simulink model "QuadSimulationVrepHoverDIV5"  (R2013a)
settings: Solver=ode1  StartTime=0  StopTime=10  FixedStep=0.01  MaxStep=0.06  RelTol=1e-3
model workspace (MAT data in the model file):
  Sig = Simulink.Signal
  Sig.DataType = 'auto'
  Sig.Dimensions = -1
  Sig.DimensionsMode = 'auto'
  Sig.Complexity = 'auto'
  Sig.SampleTime = -1
  Sig.SamplingMode = 'auto'
values from neighbouring files (symbols this model uses):
  IC = struct('P',(P),'Q',(Q),'R',(R),'Phi',(Phi),'The',(The),'Psi',(Psi),     'U',(U),'V',(V),'W',(W),'X',(X),'Y',(Y),'Z',(Z),'w1',(w1),'w2',(w2),'w3',(w3),'w4',(w4))    [ICgen.m]    (also in quadcopterDynamicsSFunction.m = block.DialogPrm(2).Data; quadcopterDynamicsSFunctionVrepV4.m = block.DialogPrm(2).Data; quadcopterDynamicsSFunctionVrepV5.m = block.DialogPrm(2).Data; quadcopterDynamicsSFunctionVrepV6.m = block.DialogPrm(2).Data)
  quadModel = struct('g',(g),'d',(d),'mass',(mass),'ct',(ct),'cq',(cq),     'Jx',(Jx),'Jy',(Jy),'Jz',(Jz),'Jm',(Jm),'Jb',(Jb),'Jbinv',(Jbinv),'dctcq',(dctcq),     'motor_m',(motor_m),'motor_dm',(motor_dm),'motor_h',(motor_h),'motor_r',(motor_r),     'ESC_m',(ESC_m),'ESC_a',(ESC_a),'ESC_b',(ESC_b),'ESC_ds',(ESC_ds),     'HUB_m',(HUB_m),'HUB_r',(HUB_r),'HUB_H',(HUB_H),     'arms_m',(arms_m),'arms_r',(arms_r),'arm ...(+111 chars)    [ModelGen.m]
undefined symbols (not defined in the file or in its folder): DiscIntNeverNeededParam, sigbuilder_block
libraries: simulink x7
Description:
  | This is a configurable quadcopter simulation.
  | This Simulink model demonstates attitude control.
  | 
  | Additional quadcopter modeling and simulation materials available at:
  | github.com/dch33/Quad-Sim
  | 
  | Copyright (C) 2014 D. Hartman, K. Landis, S. Moreno, J. Kim, M. Mehrer
  | 
  | License:
  |     This program is free software: you can redistribute it and/or modify
  |     it under the terms of the GNU LESSER GENERAL PUBLIC LICENSE as published by
  |     the Free Software Foundation, either version 3 of the License, or
  |     (at your option) any later version.
  | 
  |     This program is distributed in the hope that it will be useful,
  |     but WITHOUT ANY WARRANTY; without even the implied warranty of
  |     MERCHANTABILITY or FITNESS FOR A PARTICULAR PURPOSE.  See the
  |     GNU General Public License for more details.
  | 
  |     You should have received a copy of the GNU LESSER GENERAL PUBLIC LICENSE
  |     along with this program.  If not, see <http://www.gnu.org/licenses/>.
settings Model: ModifiedComment=Javid -- Tue Dec 01 00:24:24 2015 -- Version 1.43  Creator=David Hartman  LastModifiedBy=Javid
settings Model: ModifiedHistory=|
  | Javid -- Tue Dec 01 00:24:24 2015 -- Version 1.43
  | 
  | 
  | Javid -- Tue Dec 01 00:24:24 2015 -- Version 1.43
  | 
  | 
  | Javid -- Mon Nov 30 23:34:52 2015 -- Version 1.40
  | 
  | 
  | Javid -- Mon Nov 30 23:34:54 2015 -- Version 1.41
  | 
  | 
  | Javid -- Mon Nov 30 23:34:52 2015 -- Version 1.40
  | 
  | 
  | Cavid -- Mon Nov 30 13:04:43 2015 -- Version 1.39
  | 
  | 
  | Cavid -- Mon Nov 30 13:00:14 2015 -- Version 1.38
  | 
  | 
  | Javid -- Mon Nov 30 00:31:13 2015 -- Version 1.37
  | 
  | 
  | Javid -- Sun Nov 29 23:37:43 2015 -- Version 1.36
  | 
  | 
  | Javid -- Sun Nov 29 22:57:34 2015 -- Version 1.35
  | 
  | 
  | Javid -- Sun Nov 29 15:59:30 2015 -- Version 1.34
  | 
  | 
  | Javid -- Thu Nov 19 09:09:11 2015 -- Version 1.33
  | 
  | 
  | Javid -- Thu Nov 19 02:22:34 2015 -- Version 1.32
  | 
  | 
  | Javid -- Thu Nov 19 02:17:10 2015 -- Version 1.31
  | 
  | 
  | Javid -- Thu Nov 19 01:41:29 2015 -- Version 1.30
  | 
  | 
  | Javid -- Thu Nov 19 01:37:38 2015 -- Version 1.29
  | 
  | 
  | Javid -- Thu Nov 19 00:11:49 2015 -- Version 1.28
  | 
  | 
  | Javid -- Wed Nov 18 23:13:28 2015 -- Version 1.27
  | 
  | 
  | Javid -- Wed Nov 18 22:55:25 2015 -- Version 1.26
  | 
  | 
  | Javid -- Wed Nov 18 22:55:20 2015 -- Version 1.25
  | 
  | 
  | Javid -- Wed Nov 18 22:55:20 2015 -- Version 1.25
  | 
  | 
  | Javid -- Tue Nov 17 23:07:53 2015 -- Version 1.24
  | 
  | 
  | Javid -- Tue Nov 17 22:43:13 2015 -- Version 1.23
  | 
  | 
  | Javid -- Tue Nov 17 22:37:48 2015 -- Version 1.22
  | 
  | 
  | Javid -- Tue Nov 17 22:19:46 2015 -- Version 1.21
  | 
  | 
  | Javid -- Sun Nov 15 18:42:45 2015 -- Version 1.20
  | 
  | 
  | Javid -- Sat Nov 14 16:44:47 2015 -- Version 1.19
  | 
  | 
  | Cavid -- Mon Nov 09 15:07:19 2015 -- Version 1.18
  | 
  | 
  | Cavid -- Mon Nov 09 12:56:30 2015 -- Version 1.17
  | 
  | 
  | Javid -- Thu Nov 05 21:32:59 2015 -- Version 1.16
  | 
  | 
  | Javid -- Thu Nov 05 00:31:36 2015 -- Version 1.14
  | 
  | 
  | Javid -- Thu Nov 05 00:31:37 2015 -- Version 1.14
  | 
  | 
  | Javid -- Wed Nov 04 23:11:59 2015 -- Version 1.13
  | 
  | 
  | Javid -- Sat Oct 31 23:55:35 2015 -- Version 1.12
  | 
  | 
  | Javid -- Sat Oct 31 20:30:45 2015 -- Version 1.11
  | 
  | 
  | Cavid -- Mon Oct 19 16:53:56 2015 -- Version 1.10
  | 
  | 
  | Cavid -- Mon Oct 19 11:55:21 2015 -- Version 1.9
  | 
  | 
  | Cavid -- Mon Oct 19 11:50:10 2015 -- Version 1.8
  | 
  | 
  | Cavid -- Mon Oct 19 11:48:50 2015 -- Version 1.7
  | 
  | 
  | Cavid -- Mon Oct 19 11:27:32 2015 -- Version 1.6
  | 
  | 
  | davidhartman -- Fri Jun 06 23:19:51 2014 -- Version 1.5
  | 
  | 
  | davidhartman -- Fri Jun 06 22:53:10 2014 -- Version 1.3
settings SolverCC: AutoInsertRateTranBlk=on
settings DataIOCC: LimitDataPoints=off  SignalLogging=off
settings OptimizationCC: InlineParams=on
settings DebuggingCC: UniqueDataStoreMsg=warning  StrictBusMsg=WarnOnBusTreatedAsVector

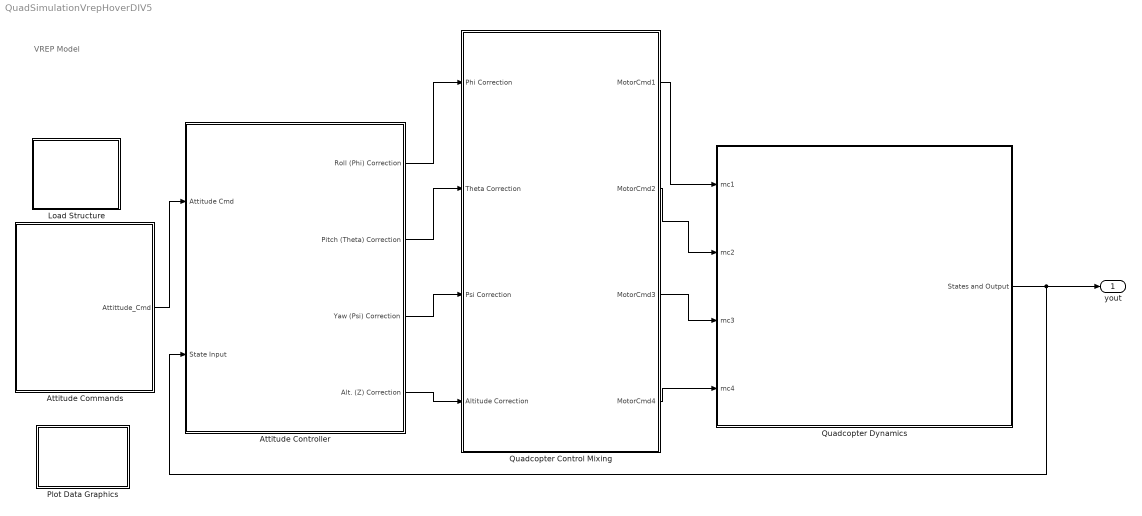
== system QuadSimulationVrepHoverDIV5 ==
  note: VREP Model
  Attitude Commands : Subsystem
  Attitude Controller : Subsystem
  Load Structure : Subsystem
      settings: OpenFcn=|
      | uiopen('load')
      | if (exist('IC')==1 && exist('quadModel')==1)
      | set_param(bdroot, 'SimulationCommand', 'update')
      | end
      mask Display: fprintf('LOAD:\nModel and\nIC\n');
  Plot Data Graphics : Subsystem
      settings: OpenFcn=|
      | if exist('yout')
      | yout = evalin('base', 'yout');
      | tout = evalin('base', 'tout');
      | quadPlotsV3(yout, tout)
      | else
      | msgbox('Simulation must be run before data can be plotted.')
      | end
      mask Display: fprintf('Plots')
  Quadcopter Control Mixing : Subsystem
      mask Display:
      | modelLoaded = evalin('base','exist(''quadModel'',''var'')');
      | if (modelLoaded==1)
      |     if (evalin('base','quadModel.plusConfig'))
      |     fprintf([' \n' ' \n'  'Configuration "+"']);
      |     else if (~evalin('base','quadModel.plusConfig'))
      |         fprintf([' \n' ' \n' 'Configuration "X"']);
      |         end
      |     end
      | else
      |     fprintf([' \n' ' \n'  'Model Not Loaded']);
      | end
  Quadcopter Dynamics : Subsystem
  yout : Outport
  wires:
  Quadcopter Control Mixing/1(MotorCmd1) -> Quadcopter Dynamics/1(mc1)
  Quadcopter Control Mixing/2(MotorCmd2) -> Quadcopter Dynamics/2(mc2)
  Quadcopter Control Mixing/3(MotorCmd3) -> Quadcopter Dynamics/3(mc3)
  Quadcopter Control Mixing/4(MotorCmd4) -> Quadcopter Dynamics/4(mc4)
  Attitude Controller/1(Roll (Phi) Correction) -> Quadcopter Control Mixing/1(Phi Correction)
  Attitude Controller/2(Pitch (Theta) Correction) -> Quadcopter Control Mixing/2(Theta Correction)
  Attitude Controller/3(Yaw (Psi) Correction) -> Quadcopter Control Mixing/3(Psi Correction)
  Attitude Controller/4(Alt. (Z) Correction) -> Quadcopter Control Mixing/4(Altitude Correction)
  Attitude Commands/1(Attittude_Cmd) -> Attitude Controller/1(Attitude Cmd)
  Quadcopter Dynamics/1(States and Output) -> Attitude Controller/2(State Input), yout/1

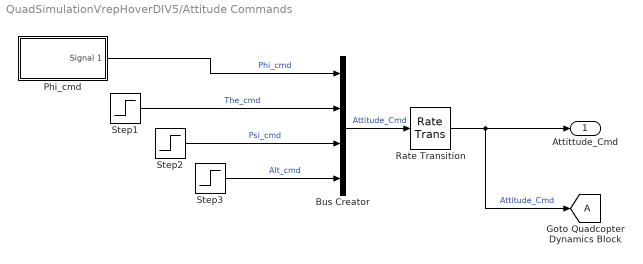
== system QuadSimulationVrepHoverDIV5/Attitude Commands ==
  Bus Creator : BusCreator
  Phi_cmd : Subsystem  Tag=STV Subsys  LoadFcn=sigbuilder_block('load');  StartFcn=sigbuilder_block('start');  StopFcn=sigbuilder_block('stop');  ClipboardFcn=sigbuilder_block('clipboard');  mask(Sigbuilder block){}
      mask help: Simulink:masks:SigbuilderBlock_MD
      mask init:
      | if ~strcmp(get_param(bdroot(gcbh),'SimulationStatus'),'stopped') tuvar = sigbuilder_block('maskInit'); end
      settings: CopyFcn=sigbuilder_block('copy');  DeleteFcn=sigbuilder_block('delete');  ModelCloseFcn=sigbuilder_block('modelClose');  PreSaveFcn=sigbuilder_block('preSave');  PauseFcn=sigbuilder_block('pause');  ContinueFcn=sigbuilder_block('continue');  NameChangeFcn=sigbuilder_block('namechange');  OpenFcn=sigbuilder_block('open',[6.75 6.75 1138.5 568.5 ]);  CloseFcn=sigbuilder_block('close');
      mask Display: plot(0, 0, 100, 100,[2, 2, 32, 32, 2], [68, 8, 8, 68, 68],[32, 2], [38, 38], [32, 19, 2],[53, 60, 44], [32, 17, 17, 2],[16, 16, 31, 31]);txt = getActiveGroup(gcbh);text(2, 100, txt,'verticalAlignment', 'top');
  Rate Transition : RateTransition  Deterministic=off  OutPortSampleTime=0.01
  Step1 : Step  Time=0  After=0  SampleTime=0
  Step2 : Step  Time=0  Before=-pi/2  After=-pi/2  SampleTime=0
  Step3 : Step  Time=0  Before=1.5  After=1.5  SampleTime=0
  Attittude_Cmd : Outport
  tag scope: A=global
  wires:
  Step3/1 -> Bus Creator/4  "Alt_cmd"
  Step2/1 -> Bus Creator/3  "Psi_cmd"
  Step1/1 -> Bus Creator/2  "The_cmd"
  Phi_cmd/1(Signal 1) -> Bus Creator/1  "Phi_cmd"
  Bus Creator/1 -> Rate Transition/1  "Attitude_Cmd"
  Rate Transition/1 -> [A], Attittude_Cmd/1  "Attitude_Cmd"

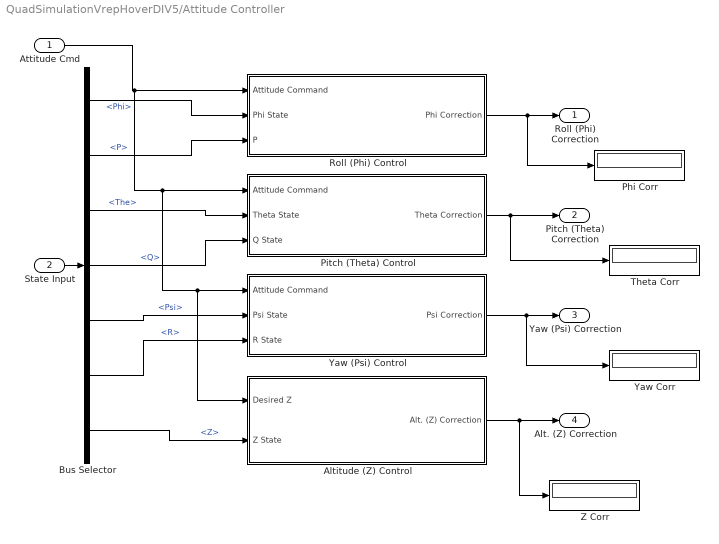
== system QuadSimulationVrepHoverDIV5/Attitude Controller ==
  Attitude Cmd : Inport
  State Input : Inport  Port=2
  Altitude (Z) Control : Subsystem  mask{Kpz=16, Kiz=1, Kdz=10, LimitOutput=on, USat=1, LSat=-1, GOffset=(sqrt((quadModel.mass*quadModel.g)/(4*quadModel.ct))-quadModel.b)/quadModel.cr}
      mask prompts: Kpz "Kp"; Kiz "Ki"; Kdz "Kd"; LimitOutput "Integral Saturation?"; USat "Upper saturation limit:"; LSat "Lower saturation limit:"; GOffset "Gravity Feedforward"
      mask help:
      | Adjust PID controller gains through this mask interface, or "look under mask" for more detailed adjustments.
      |
      | Note: Gravity Offset will not appear on block face as a value until simulation is run if it is the result of a formula involving the quadcopter model parameters.
      mask TypeOptions Kpz: Kpz/Gain
      mask TypeOptions Kiz: Kiz/Gain
      mask TypeOptions Kdz: Kdz/Gain
      mask TypeOptions LimitOutput:
      | Integrator
      | Limited/LimitOutput
      mask TypeOptions USat:
      | Integrator
      | Limited/UpperSaturationLimit
      mask TypeOptions LSat:
      | Integrator
      | Limited/LowerSaturationLimit
      mask TypeOptions GOffset: Gravity Offset (Level Flight)/Value
      mask Display:
      | fprintf(['Gravity Offset = ' num2str(GOffset) '\n' ...
      |     'Kp = ' num2str(Kpz) '\n' ...
      |     'Ki = ' num2str(Kiz) '\n' ...
      |     'Kd = ' num2str(Kdz) '\n' ...
      |     'Integral Saturation: ' LimitOutput]);
      | if strcmp(LimitOutput,'on')
      |     fprintf([' \n' ' \n' ' \n' ' \n' ' \n' '\n' ...
      |         'Limits: ' num2str(USat) ' to ' num2str(LSat)]);
      | end
  Bus Selector : BusSelector  OutputSignals=Phi,P,The,Q,Psi,R,Z
  Phi Corr : Display
  Pitch (Theta) Control : Subsystem  mask{Kpt=25, Kit=0, Kdt=6, Kdt2=0, LimitOutput=on, USat=10, LSat=-10}
      mask prompts: Kpt "Kp"; Kit "Ki"; Kdt "Kd"; Kdt2 "Kd2"; LimitOutput "Integral Saturation?"; USat "Upper saturation limit:"; LSat "Lower saturation limit:"
      mask help: Adjust PID controller gains through this mask interface, or "look under mask" for more detailed adjustments.
      mask TypeOptions Kpt: Kpt/Gain
      mask TypeOptions Kit: Kit/Gain
      mask TypeOptions Kdt: Kdt/Gain
      mask TypeOptions Kdt2: Kdt2/Gain
      mask TypeOptions LimitOutput:
      | Discrete-Time
      | Integrator/LimitOutput
      mask TypeOptions USat:
      | Discrete-Time
      | Integrator/UpperSaturationLimit
      mask TypeOptions LSat:
      | Discrete-Time
      | Integrator/LowerSaturationLimit
      mask Display:
      | % port_label('input',1,'Theta Command');
      | % port_label('input',2,'Theta State');
      | % port_label('input',3,'Q State');
      | % port_label('output',1,'Theta Correction');
      | fprintf(['Kp = ' num2str(Kpt) '\n' ...
      |     'Ki = ' num2str(Kit) '\n' ...
      |     'Kd = ' num2str(Kdt) '\n' ...
      |     'Kd2= ' num2str(Kdt2) '\n' ...
      |     'Integral Saturation: ' LimitOutput]);
      | if strcmp(LimitOutput,'on')
      |     fprintf([' \n' ' \n' ' \n' ' \n' '\n' '\n' ...
      |         'Limits: ' num2str(USat) ' to ' num2str(LSat)]);
      | end
  "Roll (Phi) Control " : Subsystem  mask{Kpp=25, Kip=0, Kdp=6, Kdp2=0, LimitOutput=on, USat=10, LSat=-10}
      mask prompts: Kpp "Kp"; Kip "Ki"; Kdp "Kd"; Kdp2 "Kd2"; LimitOutput "Integral Saturation:"; USat "Upper saturation limit:"; LSat "Lower saturation limit:"
      mask help:
      | Adjust PID controller gains through this mask interface, or "look under mask"
      | for more detailed adjustments.
      mask TypeOptions Kpp: Kpp/Gain
      mask TypeOptions Kip: Kip/Gain
      mask TypeOptions Kdp: Kdp/Gain
      mask TypeOptions Kdp2: Kdp2/Gain
      mask TypeOptions LimitOutput:
      | Discrete-Time
      | Integrator/LimitOutput
      mask TypeOptions USat:
      | Discrete-Time
      | Integrator/UpperSaturationLimit
      mask TypeOptions LSat:
      | Discrete-Time
      | Integrator/LowerSaturationLimit
      mask Display:
      | fprintf(['Kp = ' num2str(Kpp) '\n' ...
      |     'Ki = ' num2str(Kip) '\n' ...
      |     'Kd = ' num2str(Kdp) '\n'...
      |     'Kd2= ' num2str(Kdp2) '\n'...
      |     'Integral Saturation: ' LimitOutput]);
      | if strcmp(LimitOutput,'on')
      |     fprintf([' \n' ' \n' ' \n' ' \n' '\n' '\n' ...
      |         'Limits: ' num2str(USat) ' to ' num2str(LSat)]);
      | end
  Theta Corr : Display
  Yaw (Psi) Control : Subsystem  mask{Kps=0, Kis=0, Kds=0, Kds2=0, LimitOutput=on, USat=1, LSat=-1}
      mask prompts: Kps "Kp"; Kis "Ki"; Kds "Kd"; Kds2 "Kd2"; LimitOutput "Integral Saturation?"; USat "Upper saturation limit:"; LSat "Lower saturation limit:"
      mask help: Adjust PID controller gains through this mask interface, or "look under mask" for more detailed adjustments.
      mask TypeOptions Kps: Kps/Gain
      mask TypeOptions Kis: Kit/Gain
      mask TypeOptions Kds: Kds/Gain
      mask TypeOptions Kds2: Kds2/Gain
      mask TypeOptions LimitOutput:
      | Discrete-Time
      | Integrator/LimitOutput
      mask TypeOptions USat:
      | Discrete-Time
      | Integrator/UpperSaturationLimit
      mask TypeOptions LSat:
      | Discrete-Time
      | Integrator/LowerSaturationLimit
      mask Display:
      | fprintf(['Kp = ' num2str(Kps) '\n' ...
      |     'Ki = ' num2str(Kis) '\n' ...
      |     'Kd = ' num2str(Kds) '\n' ...
      |     'Kd2 = ' num2str(Kds2) '\n' ...
      |     'Integral Saturation: ' LimitOutput]);
      | if strcmp(LimitOutput,'on')
      |     fprintf([' \n' ' \n' ' \n' ' \n' '\n' '\n' ...
      |         'Limits: ' num2str(USat) ' to ' num2str(LSat)]);
      | end
  Yaw Corr : Display
  Z Corr : Display
  Roll (Phi) Correction : Outport
  Pitch (Theta) Correction : Outport  Port=2
  Yaw (Psi) Correction : Outport  Port=3
  Alt. (Z) Correction : Outport  Port=4
  wires:
  Bus Selector/6 -> Yaw (Psi) Control/3(R State)  "<R>"
  Bus Selector/4 -> Pitch (Theta) Control/3(Q State)  "<Q>"
  Bus Selector/2 -> "Roll (Phi) Control "/3(P)  "<P>"
  Bus Selector/3 -> Pitch (Theta) Control/2(Theta State)  "<The>"
  Bus Selector/7 -> Altitude (Z) Control/2(Z State)  "<Z>"
  Bus Selector/5 -> Yaw (Psi) Control/2(Psi State)  "<Psi>"
  Yaw (Psi) Control/1(Psi Correction) -> Yaw Corr/1, Yaw (Psi) Correction/1
  Pitch (Theta) Control/1(Theta Correction) -> Theta Corr/1, Pitch (Theta) Correction/1
  Bus Selector/1 -> "Roll (Phi) Control "/2(Phi State)  "<Phi>"
  "Roll (Phi) Control "/1(Phi Correction) -> Phi Corr/1, Roll (Phi) Correction/1
  Altitude (Z) Control/1(Alt. (Z) Correction) -> Z Corr/1, Alt. (Z) Correction/1
  State Input/1 -> Bus Selector/1
  Attitude Cmd/1 -> "Roll (Phi) Control "/1("Attitude Command "), Pitch (Theta) Control/1(Attitude Command), Yaw (Psi) Control/1(Attitude Command), Altitude (Z) Control/1(Desired Z)

== system QuadSimulationVrepHoverDIV5/Load Structure ==

== system QuadSimulationVrepHoverDIV5/Plot Data Graphics ==

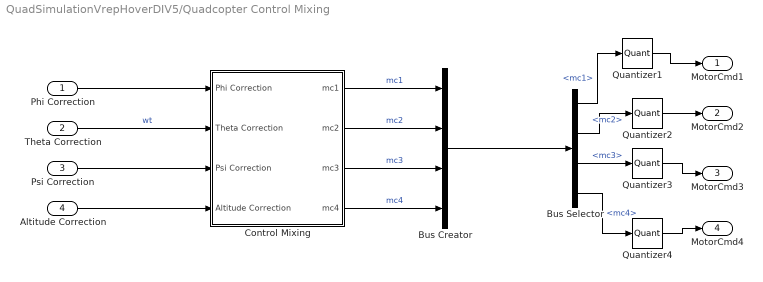
== system QuadSimulationVrepHoverDIV5/Quadcopter Control Mixing ==
  Phi Correction : Inport
  Theta Correction : Inport  Port=2
  Psi Correction : Inport  Port=3
  Altitude Correction : Inport  Port=4
  Bus Creator : BusCreator
  Bus Selector : BusSelector  OutputSignals=mc1,mc2,mc3,mc4
  Control Mixing : Subsystem
  "Quantizer1 " : Quantizer  QuantizationInterval=0.1
  "Quantizer2 " : Quantizer  QuantizationInterval=0.1
  Quantizer3 : Quantizer  QuantizationInterval=0.1
  "Quantizer4 " : Quantizer  QuantizationInterval=0.1
  MotorCmd1 : Outport
  MotorCmd2 : Outport  Port=2
  MotorCmd3 : Outport  Port=3
  MotorCmd4 : Outport  Port=4
  wires:
  Bus Creator/1 -> Bus Selector/1
  Control Mixing/4(mc4) -> Bus Creator/4  "mc4"
  Control Mixing/3(mc3) -> Bus Creator/3  "mc3"
  Control Mixing/2(mc2) -> Bus Creator/2  "mc2"
  Control Mixing/1(mc1) -> Bus Creator/1  "mc1"
  Altitude Correction/1 -> Control Mixing/4(Altitude Correction)
  Psi Correction/1 -> Control Mixing/3(Psi Correction)
  Theta Correction/1 -> Control Mixing/2(Theta Correction)  "wt"
  Phi Correction/1 -> Control Mixing/1(Phi Correction)
  Bus Selector/1 -> "Quantizer1 "/1  "<mc1>"
  "Quantizer1 "/1 -> MotorCmd1/1
  Bus Selector/2 -> "Quantizer2 "/1  "<mc2>"
  "Quantizer2 "/1 -> MotorCmd2/1
  Bus Selector/3 -> Quantizer3/1  "<mc3>"
  Quantizer3/1 -> MotorCmd3/1
  Bus Selector/4 -> "Quantizer4 "/1  "<mc4>"
  "Quantizer4 "/1 -> MotorCmd4/1

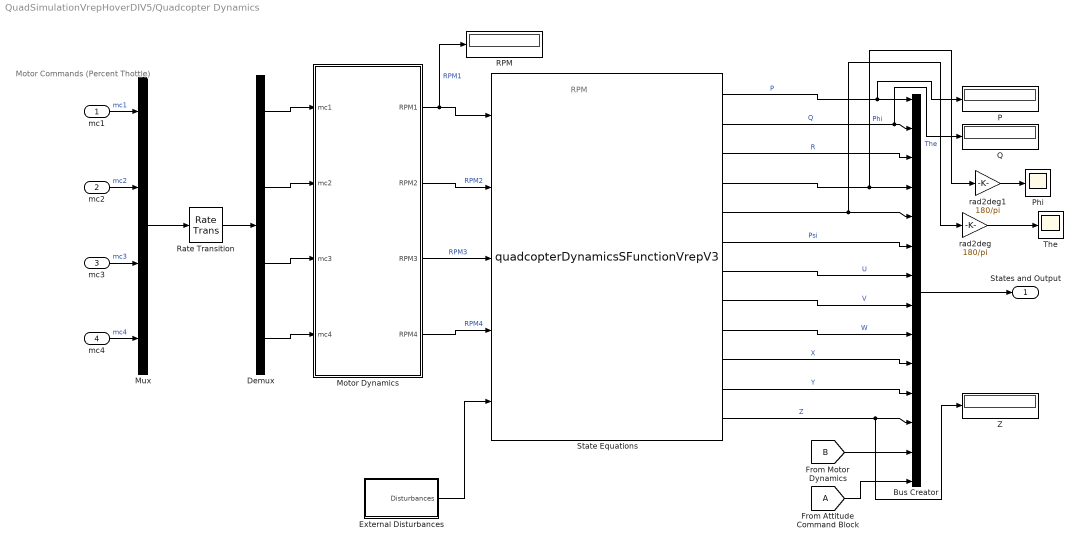
== system QuadSimulationVrepHoverDIV5/Quadcopter Dynamics ==
  note: Motor Commands
      | (Percent Thottle)
  note: RPM
  mc1 : Inport
  mc2 : Inport  Port=2
  mc3 : Inport  Port=3
  mc4 : Inport  Port=4
  Bus Creator : BusCreator  Inputs='P','Q','R','Phi','The','Psi','U','V','W','X','Y','Z','mc and RPM','Attitude_Cmd'
  Demux : Demux
  External Disturbances : Subsystem
  Motor Dynamics : Subsystem
  Mux : Mux
  P : Display
  Phi : Scope
  Q : Display
  RPM : Display
  Rate Transition : RateTransition  Deterministic=off  OutPortSampleTime=0.01
  State Equations : M-S-Function  FunctionName=quadcopterDynamicsSFunctionVrepV3  Parameters=quadModel, IC
      mask Display:
      | port_label('input', 1, 'RPM1')
      | port_label('input', 2, 'RPM2')
      | port_label('input', 3, 'RPM3')
      | port_label('input', 4, 'RPM4')
      | port_label('input', 5, 'Disturbances')
      | port_label('output', 1, 'P')
      | port_label('output', 2, 'Q')
      | port_label('output', 3, 'R')
      | port_label('output', 4, 'Phi')
      | port_label('output', 5, 'The')
      | port_label('output', 6, 'Psi')
      | port_label('output', 7, 'U')
      | port_label('output', 8, 'V')
      | port_label('output', 9, 'W')
      | port_label('output', 10, 'X')
      | port_label('output', 11, 'Y')
      | port_label('output', 12, 'Z')
  The : Scope
  Z : Display
  rad2deg : Gain  Gain=180/pi
  rad2deg1 : Gain  Gain=180/pi
  States and Output : Outport
  wires:
  External Disturbances/1("Disturbances ") -> State Equations/5
  Motor Dynamics/4(RPM4) -> State Equations/4  "RPM4"
  Motor Dynamics/3(RPM3) -> State Equations/3  "RPM3"
  Motor Dynamics/2(RPM2) -> State Equations/2  "RPM2"
  Motor Dynamics/1(RPM1) -> RPM/1, State Equations/1  "RPM1"
  State Equations/12 -> Z/1, Bus Creator/12  "Z"
  State Equations/11 -> Bus Creator/11  "Y"
  State Equations/10 -> Bus Creator/10  "X"
  State Equations/9 -> Bus Creator/9  "W"
  State Equations/8 -> Bus Creator/8  "V"
  State Equations/7 -> Bus Creator/7  "U"
  State Equations/6 -> Bus Creator/6  "Psi"
  State Equations/5 -> rad2deg/1, Bus Creator/5  "The"
  State Equations/4 -> rad2deg1/1, Bus Creator/4  "Phi"
  State Equations/3 -> Bus Creator/3  "R"
  State Equations/2 -> Q/1, Bus Creator/2  "Q"
  State Equations/1 -> P/1, Bus Creator/1  "P"
  rad2deg/1 -> The/1
  rad2deg1/1 -> Phi/1
  mc1/1 -> Mux/1  "mc1"
  mc2/1 -> Mux/2  "mc2"
  mc3/1 -> Mux/3  "mc3"
  mc4/1 -> Mux/4  "mc4"
  Mux/1 -> Rate Transition/1
  Rate Transition/1 -> Demux/1
  Demux/1 -> Motor Dynamics/1(mc1)
  Demux/2 -> Motor Dynamics/2(mc2)
  Demux/3 -> Motor Dynamics/3(mc3)
  Demux/4 -> Motor Dynamics/4(mc4)
  [B] -> Bus Creator/13
  [A] -> Bus Creator/14
  Bus Creator/1 -> States and Output/1

== system QuadSimulationVrepHoverDIV5/Attitude Commands/Phi_cmd ==
  Demux : Demux  Tag=STV Demux  Outputs=1
  FromWs : FromWorkspace  Tag=STV FromWs  VariableName=tuvar  SampleTime=0
      SigBuilderData=|
      | common.afterFinalStr = 'Extrapolate'
      | common.sampleTime = 0
      | dataSet.timeRange = [0 10]
      | dataSet.name = 'Group 1'
      | sbobj.Groups.Name = 'Group 1'
      | sbobj.Groups.Signals.Name = 'Signal 1'
      | sbobj.Groups.Signals.XData = [0 1 1.36 1.64 1.66 1.84 2 3.62 3.76 4 4.44 4.48 10]
      | sbobj.Groups.Signals.YData = [0 0 -0.282743338823 -0.2835 -0.523599822796 -0.523 0 0 0.314159265359 0.518362787842 0.52 0 0]
  Signal 1 : Outport  Tag=STV Outport
  wires:
  Demux/1 -> Signal 1/1
  FromWs/1 -> Demux/1

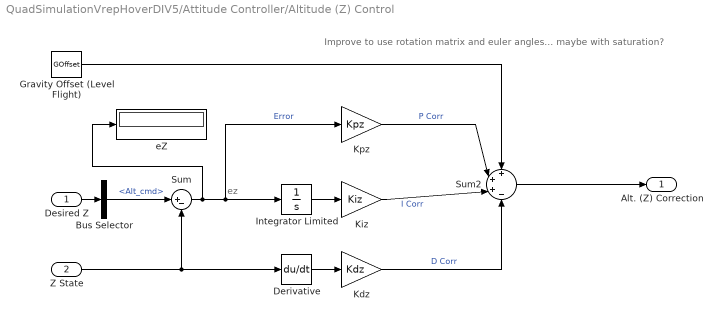
== system QuadSimulationVrepHoverDIV5/Attitude Controller/Altitude (Z) Control ==
  note: ez
  note: Improve to use rotation matrix and euler angles...
      | maybe with saturation?
  Desired Z : Inport
  Z State : Inport  Port=2
  Bus Selector : BusSelector  OutputSignals=Alt_cmd
  Derivative : Derivative
  Gravity Offset (Level Flight) : Constant  Value=GOffset
  Integrator Limited : Integrator  LimitOutput=on  UpperSaturationLimit=USat  LowerSaturationLimit=LSat
  Kdz : Gain  Gain=Kdz
  Kiz : Gain  Gain=Kiz
  Kpz : Gain  Gain=Kpz
  Sum : Sum  Inputs=|+-
  Sum2 : Sum  Inputs=+++-
  eZ : Display
  Alt. (Z) Correction : Outport
  wires:
  Derivative/1 -> Kdz/1
  Bus Selector/1 -> Sum/1  "<Alt_cmd>"
  Integrator Limited/1 -> Kiz/1
  Kdz/1 -> Sum2/4  "D Corr"
  Kiz/1 -> Sum2/3  "I Corr"
  Sum/1 -> eZ/1, Kpz/1, Integrator Limited/1  "Error"
  Kpz/1 -> Sum2/2  "P Corr"
  Sum2/1 -> Alt. (Z) Correction/1
  Z State/1 -> Sum/2, Derivative/1
  Desired Z/1 -> Bus Selector/1
  Gravity Offset (Level Flight)/1 -> Sum2/1

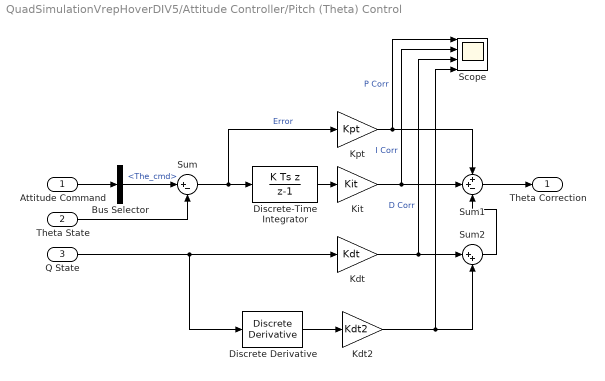
== system QuadSimulationVrepHoverDIV5/Attitude Controller/Pitch (Theta) Control ==
  Attitude Command : Inport
  Theta State : Inport  Port=2
  Q State : Inport  Port=3
  Bus Selector : BusSelector  OutputSignals=The_cmd
  Discrete Derivative : simulink/Discrete/Discrete Derivative  gainval=1.0  ICPrevScaledInput=0.0  InputProcessing=Inherited  OutMin=[]  OutMax=[]  OutDataType=fixdt(1, 16)  OutScaling=2^-10  DoSatur=off
  Discrete-Time Integrator : DiscreteIntegrator  IntegratorMethod=Integration: Backward Euler  SampleTime=0.01  LimitOutput=on  UpperSaturationLimit=USat  LowerSaturationLimit=LSat  ICPrevOutput=DiscIntNeverNeededParam  ICPrevScaledInput=DiscIntNeverNeededParam
  Kdt : Gain  Gain=Kdt
  Kdt2 : Gain  Gain=Kdt2
  Kit : Gain  Gain=Kit
  Kpt : Gain  Gain=Kpt
  Scope : Scope  NumInputPorts=4
      settings: ShowLegends=on  YMin=-0.12~0.0775~-0.125~-0.4  YMax=-0.025~0.1075~0.25~0.3  SaveName=ScopeData2
  Sum : Sum  Inputs=|+-
  Sum1 : Sum  Inputs=++-
  Sum2 : Sum  Inputs=|++
  Theta Correction : Outport
  wires:
  Sum/1 -> Discrete-Time Integrator/1, Kpt/1  "Error"
  Attitude Command/1 -> Bus Selector/1
  Theta State/1 -> Sum/2
  Discrete-Time Integrator/1 -> Kit/1
  Bus Selector/1 -> Sum/1  "<The_cmd>"
  Q State/1 -> Discrete Derivative/1, Kdt/1
  Kpt/1 -> Scope/1, Sum1/1  "P Corr"
  Kit/1 -> Scope/2, Sum1/2  "I Corr"
  Sum1/1 -> Theta Correction/1
  Discrete Derivative/1 -> Kdt2/1
  Sum2/1 -> Sum1/3
  Kdt2/1 -> Sum2/2, Scope/4
  Kdt/1 -> Sum2/1, Scope/3  "D Corr"

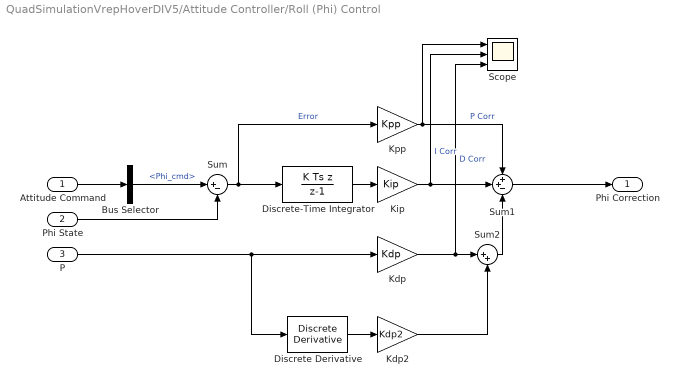
== system QuadSimulationVrepHoverDIV5/Attitude Controller/Roll (Phi) Control  ==
  "Attitude Command " : Inport
  Phi State : Inport  Port=2
  P : Inport  Port=3
  Bus Selector : BusSelector  OutputSignals=Phi_cmd
  Discrete Derivative : simulink/Discrete/Discrete Derivative  gainval=1.0  ICPrevScaledInput=0.0  InputProcessing=Inherited  OutMin=[]  OutMax=[]  OutDataType=fixdt(1, 16)  OutScaling=2^-10  DoSatur=off
  Discrete-Time Integrator : DiscreteIntegrator  IntegratorMethod=Integration: Backward Euler  SampleTime=0.01  LimitOutput=on  UpperSaturationLimit=USat  LowerSaturationLimit=LSat  ICPrevOutput=DiscIntNeverNeededParam  ICPrevScaledInput=DiscIntNeverNeededParam
  Kdp : Gain  Gain=Kdp
  Kdp2 : Gain  Gain=Kdp2
  Kip : Gain  Gain=Kip
  Kpp : Gain  Gain=Kpp
  Scope : Scope  NumInputPorts=3
      settings: ShowLegends=on  YMin=-5~-5~-5  YMax=5~5~5
  Sum : Sum  Inputs=|+-
  Sum1 : Sum  Inputs=++-
  Sum2 : Sum  Inputs=|++
  Phi Correction : Outport
  wires:
  Sum/1 -> Discrete-Time Integrator/1, Kpp/1  "Error"
  Phi State/1 -> Sum/2
  Sum1/1 -> Phi Correction/1
  Kpp/1 -> Scope/1, Sum1/1  "P Corr"
  Kdp/1 -> Sum2/1, Scope/3  "D Corr"
  Kip/1 -> Scope/2, Sum1/2  "I Corr"
  Discrete-Time Integrator/1 -> Kip/1
  "Attitude Command "/1 -> Bus Selector/1
  Bus Selector/1 -> Sum/1  "<Phi_cmd>"
  Discrete Derivative/1 -> Kdp2/1
  Kdp2/1 -> Sum2/2
  Sum2/1 -> Sum1/3
  P/1 -> Discrete Derivative/1, Kdp/1

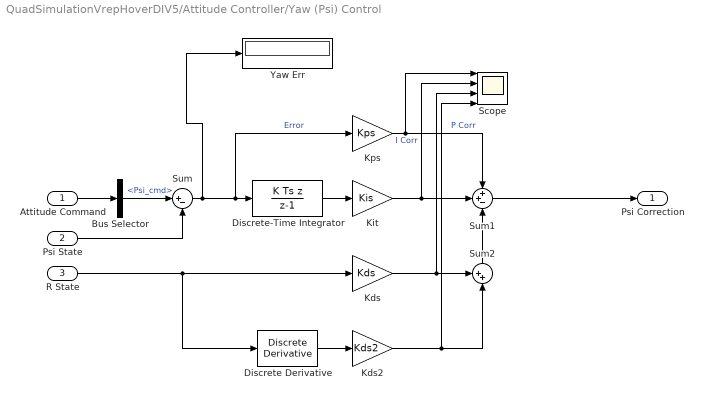
== system QuadSimulationVrepHoverDIV5/Attitude Controller/Yaw (Psi) Control ==
  Attitude Command : Inport
  Psi State : Inport  Port=2
  R State : Inport  Port=3
  Bus Selector : BusSelector  OutputSignals=Psi_cmd
  Discrete Derivative : simulink/Discrete/Discrete Derivative  gainval=1.0  ICPrevScaledInput=0.0  InputProcessing=Inherited  OutMin=[]  OutMax=[]  OutDataType=fixdt(1, 16)  OutScaling=2^-10  DoSatur=off
  Discrete-Time Integrator : DiscreteIntegrator  IntegratorMethod=Integration: Backward Euler  SampleTime=0.01  LimitOutput=on  UpperSaturationLimit=USat  LowerSaturationLimit=LSat  ICPrevOutput=DiscIntNeverNeededParam  ICPrevScaledInput=DiscIntNeverNeededParam
  Kds : Gain  Gain=Kds
  Kds2 : Gain  Gain=Kds2
  Kit : Gain  Gain=Kis
  Kps : Gain  Gain=Kps
  Scope : Scope  NumInputPorts=4
      settings: ShowLegends=on  YMin=0~0~0~0  YMax=0.65~0.004~0.00045~0.006
  Sum : Sum  Inputs=|+-
  Sum1 : Sum  Inputs=++-
  Sum2 : Sum  Inputs=++|
  "Yaw Err " : Display
  Psi Correction : Outport
  wires:
  Sum/1 -> "Yaw Err "/1, Discrete-Time Integrator/1, Kps/1  "Error"
  Attitude Command/1 -> Bus Selector/1
  Sum1/1 -> Psi Correction/1
  Psi State/1 -> Sum/2
  Kps/1 -> Scope/1, Sum1/1  "P Corr"
  Kds/1 -> Sum2/1, Scope/3
  Kit/1 -> Scope/2, Sum1/2  "I Corr"
  Discrete-Time Integrator/1 -> Kit/1
  Bus Selector/1 -> Sum/1  "<Psi_cmd>"
  R State/1 -> Discrete Derivative/1, Kds/1
  Discrete Derivative/1 -> Kds2/1
  Kds2/1 -> Scope/4, Sum2/2
  Sum2/1 -> Sum1/3

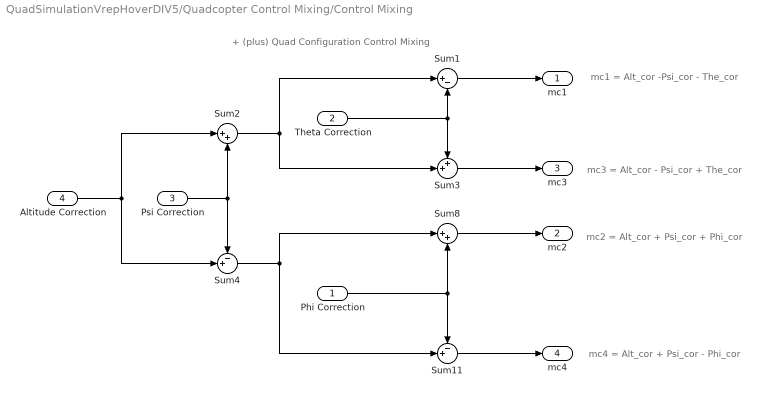
== system QuadSimulationVrepHoverDIV5/Quadcopter Control Mixing/Control Mixing ==
  note: mc1 = Alt_cor -Psi_cor - The_cor
  note: mc3 = Alt_cor - Psi_cor + The_cor
  note: mc4 = Alt_cor + Psi_cor - Phi_cor
  note: + (plus) Quad Configuration Control Mixing
  note: mc2 = Alt_cor + Psi_cor + Phi_cor
  Phi Correction : Inport
  Theta Correction : Inport  Port=2
  Psi Correction : Inport  Port=3
  Altitude Correction : Inport  Port=4
  Sum1 : Sum  Inputs=|+-
  Sum11 : Sum  Inputs=-+|
  Sum2 : Sum  Inputs=|++
  Sum3 : Sum  Inputs=++|
  Sum4 : Sum  Inputs=-+|
  Sum8 : Sum  Inputs=|++
  mc1 : Outport
  mc2 : Outport  Port=2
  mc3 : Outport  Port=3
  mc4 : Outport  Port=4
  wires:
  Sum11/1 -> mc4/1
  Sum8/1 -> mc2/1
  Sum3/1 -> mc3/1
  Sum1/1 -> mc1/1
  Phi Correction/1 -> Sum11/1, Sum8/2
  Sum4/1 -> Sum8/1, Sum11/2
  Psi Correction/1 -> Sum2/2, Sum4/1
  Sum2/1 -> Sum1/1, Sum3/2
  Altitude Correction/1 -> Sum4/2, Sum2/1
  Theta Correction/1 -> Sum3/1, Sum1/2

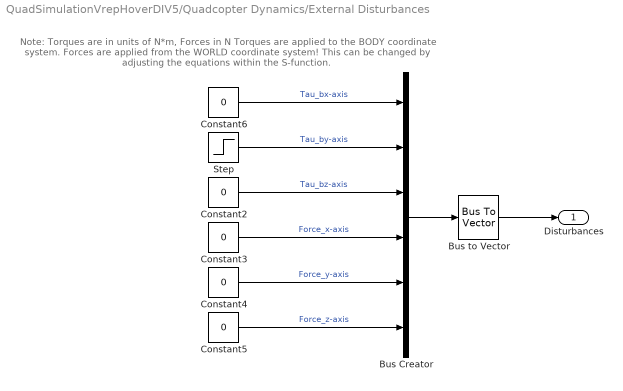
== system QuadSimulationVrepHoverDIV5/Quadcopter Dynamics/External Disturbances ==
  note: Note: Torques are in units of N*m, Forces in N
      | Torques are applied to the BODY coordinate system.
      | Forces are applied from the WORLD coordinate system!
      | This can be changed by adjusting the equations within the S-function.
  Bus Creator : BusCreator  Inputs=6
  Bus to Vector : BusToVector
  Constant{2..6} (5 alike) : Constant  Value=0
  Step : Step  After=0  SampleTime=0
  "Disturbances " : Outport
  wires:
  Constant5/1 -> Bus Creator/6  "Force_z-axis"
  Constant4/1 -> Bus Creator/5  "Force_y-axis"
  Constant3/1 -> Bus Creator/4  "Force_x-axis"
  Constant2/1 -> Bus Creator/3  "Tau_bz-axis"
  Step/1 -> Bus Creator/2  "Tau_by-axis"
  Constant6/1 -> Bus Creator/1  "Tau_bx-axis"
  Bus Creator/1 -> Bus to Vector/1
  Bus to Vector/1 -> "Disturbances "/1

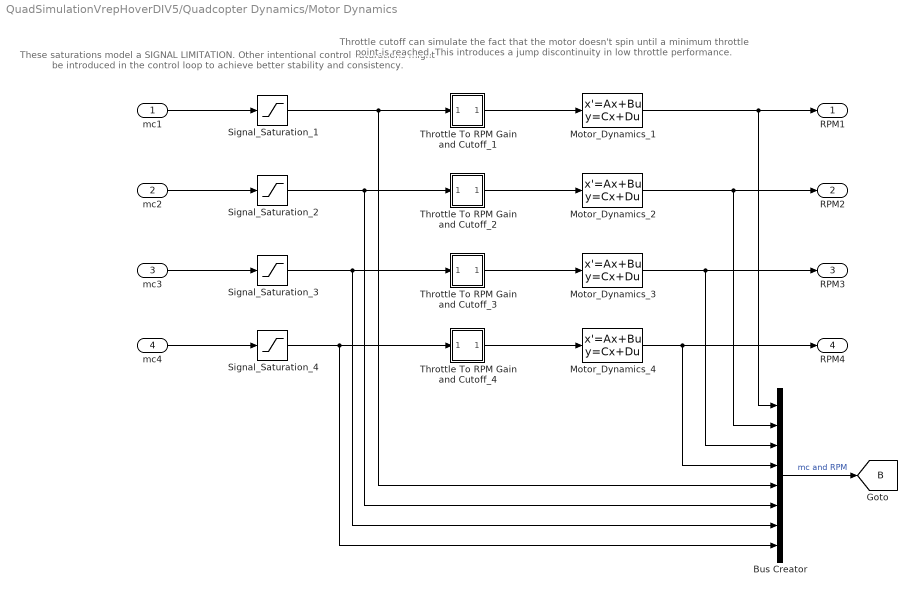
== system QuadSimulationVrepHoverDIV5/Quadcopter Dynamics/Motor Dynamics ==
  note: These saturations model a SIGNAL LIMITATION.
      | Other intentional control saturations might be introduced in the
      | control loop to achieve better stability and consistency.
  note: Throttle cutoff can simulate the fact that the motor doesn't
      | spin until a minimum throttle point is reached. This introduces
      | a jump discontinuity in low throttle performance.
  mc1 : Inport
  mc2 : Inport  Port=2
  mc3 : Inport  Port=3
  mc4 : Inport  Port=4
  Bus Creator : BusCreator  Inputs=8
  Motor_Dynamics_1 : StateSpace  A=-1/quadModel.T  C=1/quadModel.T  D=0  X0=IC.w1*quadModel.T
  Motor_Dynamics_2 : StateSpace  A=-1/quadModel.T  C=1/quadModel.T  D=0  X0=IC.w2*quadModel.T
  Motor_Dynamics_3 : StateSpace  A=-1/quadModel.T  C=1/quadModel.T  D=0  X0=IC.w3*quadModel.T
  Motor_Dynamics_4 : StateSpace  A=-1/quadModel.T  C=1/quadModel.T  D=0  X0=IC.w4*quadModel.T
  Signal_Saturation_{1..4} (4 alike) : Saturate  UpperLimit=100  LowerLimit=0
  Throttle To RPM Gain and Cutoff_1 : Subsystem
  Throttle To RPM Gain and Cutoff_2 : Subsystem
  Throttle To RPM Gain and Cutoff_3 : Subsystem
  Throttle To RPM Gain and Cutoff_4 : Subsystem
  RPM1 : Outport
  RPM2 : Outport  Port=2
  RPM3 : Outport  Port=3
  RPM4 : Outport  Port=4
  tag scope: B=global
  wires:
  Bus Creator/1 -> [B]  "mc and RPM"
  Motor_Dynamics_4/1 -> RPM4/1, Bus Creator/4
  Motor_Dynamics_3/1 -> RPM3/1, Bus Creator/3
  Motor_Dynamics_2/1 -> RPM2/1, Bus Creator/2
  Motor_Dynamics_1/1 -> RPM1/1, Bus Creator/1
  Throttle To RPM Gain and Cutoff_4/1(Out5) -> Motor_Dynamics_4/1
  Throttle To RPM Gain and Cutoff_3/1(Out5) -> Motor_Dynamics_3/1
  Throttle To RPM Gain and Cutoff_2/1(Out5) -> Motor_Dynamics_2/1
  Throttle To RPM Gain and Cutoff_1/1(Out5) -> Motor_Dynamics_1/1
  Signal_Saturation_4/1 -> Throttle To RPM Gain and Cutoff_4/1(In5), Bus Creator/8
  Signal_Saturation_3/1 -> Throttle To RPM Gain and Cutoff_3/1(In5), Bus Creator/7
  Signal_Saturation_2/1 -> Throttle To RPM Gain and Cutoff_2/1(In5), Bus Creator/6
  Signal_Saturation_1/1 -> Throttle To RPM Gain and Cutoff_1/1(In5), Bus Creator/5
  mc3/1 -> Signal_Saturation_3/1
  mc2/1 -> Signal_Saturation_2/1
  mc4/1 -> Signal_Saturation_4/1
  mc1/1 -> Signal_Saturation_1/1

== system QuadSimulationVrepHoverDIV5/Quadcopter Dynamics/Motor Dynamics/Throttle To RPM Gain and Cutoff_1 ==
  note: Output equals linearly scaled RPM
      | for given throttle input if throttle input >=Throttle Cuttoff (minThr)
      | else output is zero.
  In5 : Inport
  Constant : Constant  Value=quadModel.b
  Gain : Gain  Gain=quadModel.cr
  Minimum Throttle Cutoff : simulink/Logic and Bit Operations/Compare To Constant  relop=>=  const=quadModel.minThr  OutDataTypeStr=uint8
  Product : Product
  Sum1 : Sum  Inputs=++|
  Out5 : Outport
  wires:
  Constant/1 -> Sum1/1
  Sum1/1 -> Product/1
  Gain/1 -> Sum1/2
  In5/1 -> Minimum Throttle Cutoff/1, Gain/1
  Product/1 -> Out5/1
  Minimum Throttle Cutoff/1 -> Product/2

== system QuadSimulationVrepHoverDIV5/Quadcopter Dynamics/Motor Dynamics/Throttle To RPM Gain and Cutoff_2 ==
  note: Output equals linearly scaled RPM
      | for given throttle input if throttle input >=Throttle Cuttoff (minThr)
      | else output is zero.
  In5 : Inport
  Constant : Constant  Value=quadModel.b
  Gain : Gain  Gain=quadModel.cr
  Minimum Throttle Cutoff : simulink/Logic and Bit Operations/Compare To Constant  relop=>=  const=quadModel.minThr  OutDataTypeStr=uint8
  Product : Product
  Sum1 : Sum  Inputs=++|
  Out5 : Outport
  wires:
  Constant/1 -> Sum1/1
  Sum1/1 -> Product/1
  Gain/1 -> Sum1/2
  In5/1 -> Minimum Throttle Cutoff/1, Gain/1
  Product/1 -> Out5/1
  Minimum Throttle Cutoff/1 -> Product/2

== system QuadSimulationVrepHoverDIV5/Quadcopter Dynamics/Motor Dynamics/Throttle To RPM Gain and Cutoff_3 ==
  note: Output equals linearly scaled RPM
      | for given throttle input if throttle input >=Throttle Cuttoff (minThr)
      | else output is zero.
  In5 : Inport
  Constant : Constant  Value=quadModel.b
  Gain : Gain  Gain=quadModel.cr
  Minimum Throttle Cutoff : simulink/Logic and Bit Operations/Compare To Constant  relop=>=  const=quadModel.minThr  OutDataTypeStr=uint8
  Product : Product
  Sum1 : Sum  Inputs=++|
  Out5 : Outport
  wires:
  Constant/1 -> Sum1/1
  Sum1/1 -> Product/1
  Gain/1 -> Sum1/2
  In5/1 -> Minimum Throttle Cutoff/1, Gain/1
  Product/1 -> Out5/1
  Minimum Throttle Cutoff/1 -> Product/2

== system QuadSimulationVrepHoverDIV5/Quadcopter Dynamics/Motor Dynamics/Throttle To RPM Gain and Cutoff_4 ==
  note: Output equals linearly scaled RPM
      | for given throttle input if throttle input >=Throttle Cuttoff (minThr)
      | else output is zero.
  In5 : Inport
  Constant : Constant  Value=quadModel.b
  Gain : Gain  Gain=quadModel.cr
  Minimum Throttle Cutoff : simulink/Logic and Bit Operations/Compare To Constant  relop=>=  const=quadModel.minThr  OutDataTypeStr=uint8
  Product : Product
  Sum1 : Sum  Inputs=++|
  Out5 : Outport
  wires:
  Constant/1 -> Sum1/1
  Sum1/1 -> Product/1
  Gain/1 -> Sum1/2
  In5/1 -> Minimum Throttle Cutoff/1, Gain/1
  Product/1 -> Out5/1
  Minimum Throttle Cutoff/1 -> Product/2
